simulink model "TESTINGSIMULINKPARTC"  (R2024b)
settings: Solver=VariableStepAuto  StartTime=0.0  StopTime=6  RelTol=1e-3
settings Model: Creator=miao
settings OptimizationCC: ReuseModelBlockBuffer=off
settings RTWCC: GPUComputeCapability=3.5

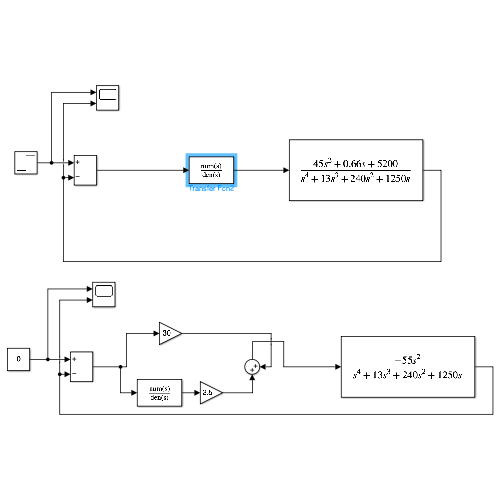
[thumbnail: Simulink's stored preview of the top-level diagram]
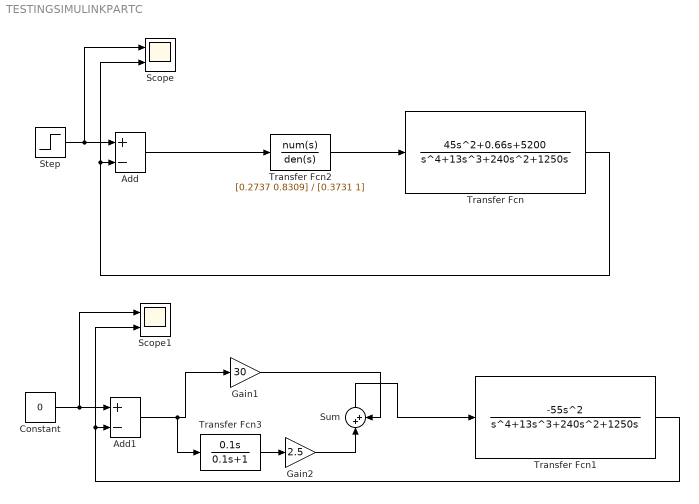
== system TESTINGSIMULINKPARTC ==
  Add : Sum  Inputs=+-
  Add1 : Sum  Inputs=+-
  Constant : Constant  Value=0
  Gain1 : Gain  Gain=30
  Gain2 : Gain  Gain=2.5
  Scope : Scope  NumInputPorts=2
  Scope1 : Scope  NumInputPorts=2
  Step : Step  SampleTime=0
  Sum : Sum  Inputs=|++
  Transfer Fcn : TransferFcn  Numerator=[45 0.66 5200]  Denominator=[1 13 240 1250 0]
  Transfer Fcn1 : TransferFcn  Numerator=[-55 0 0]  Denominator=[1 13 240 1250 0]
  Transfer Fcn2 : TransferFcn  Numerator=[0.2737 0.8309]  Denominator=[0.3731 1]
  Transfer Fcn3 : TransferFcn  Numerator=[0.1 0]  Denominator=[0.1 1]
  wires:
  Transfer Fcn2/1 -> Transfer Fcn/1
  Step/1 -> Scope/1, Add/1
  Transfer Fcn/1 -> Scope/2, Add/2
  Add1/1 -> Transfer Fcn3/1, Gain1/1
  Transfer Fcn1/1 -> Scope1/2, Add1/2
  Constant/1 -> Add1/1, Scope1/1
  Gain2/1 -> Sum/1
  Add/1 -> Transfer Fcn2/1
  Transfer Fcn3/1 -> Gain2/1
  Gain1/1 -> Sum/2
  Sum/1 -> Transfer Fcn1/1
